simulink model "mvdc_KF_PointMassSep"  (R2018b)
settings: configuration reference "Active" (kept outside this file)
undefined symbols (not defined in the file): P_VDC_enableCovPropagation, P_VDC_ManualInitializationStartPose, P_VDC_ManualInitializationStateEstimation, P_VDC_measCov_GPS, P_VDC_measCov_velocity, P_VDC_measCov_VLOC, P_VDC_OutlierBounds, P_VDC_processCovVelocityFused, P_VDC_Var_ax_mps2, P_VDC_Var_ay_mps2, P_VDC_Var_yawRate_radps, P_VDC_YawAngleDepCovMode, res_dGPS_m, res_dPsi_radps, res_dVLOC_m, res_PsiGPS_rad, res_PsiVLOC_rad, res_sGPS_m, res_sVLOC_m, res_vx_mps, res_vy_mps, res_xGPS_m, res_xVLOC_m, res_yGPS_m, res_yVLOC_m, tS
libraries: rr_general x2
settings Model: DataDictionary=mvdc_KF.sldd  Creator=Madeline  LastModifiedBy=Kappertz

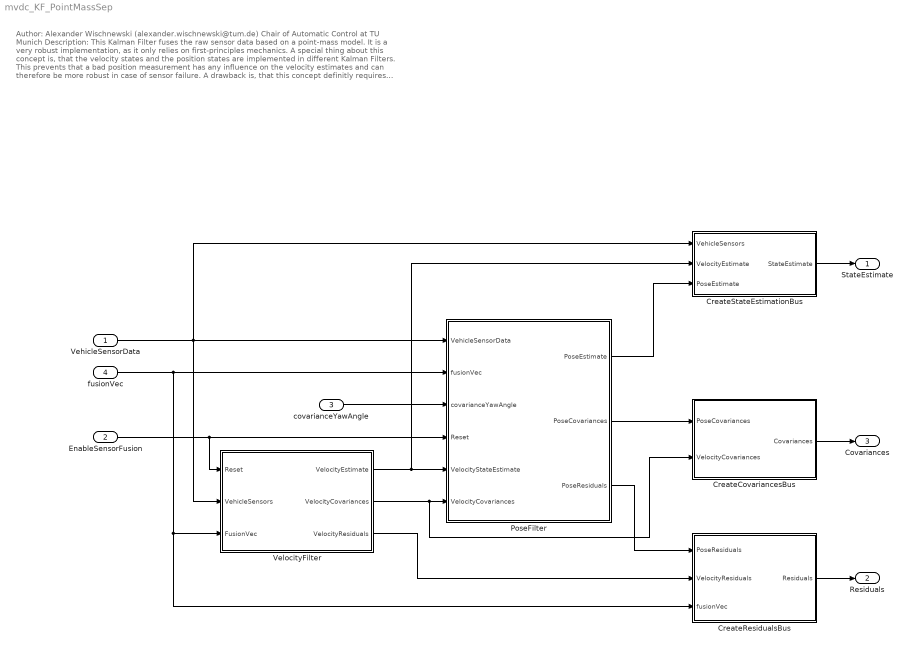
== system mvdc_KF_PointMassSep ==
  note: Author: Alexander Wischnewski (alexander.wischnewski@tum.de)
      | Chair of Automatic Control at TU Munich
      |
      | Description: This Kalman Filter fuses the raw sensor data based on a point-mass model. It is a very robust implementation, as it only relies on first-principles mechanics. A special thing about this concept is, that the velocity states and the position states are implemented in different Kalman Filters. This prevents that a bad position measurement has any influence on the velocity estimates and can therefore be more robust in case of sensor failure. A drawback is, that this concept definitly requires measurement of the vehicle-fixed velocities in lateral and longitudinal direction. Another drawback compared to a more complex vehicle model is, that it cannot filter the yaw rate as there are no derivative information about the yaw rate available. However, it is easy to tune and has comparable performance over the whole range of operating points.
      |
      | Inputs:
      | EnableSensorFusion Enable bit which activates the Kalman Filter
      | VehicleSensorData Raw sensor data
      | ActualPathOrientation Path orientation provided by the trajectory planner (used for weighting GPS and LIDAR via Covariance Matrix)
      | fusionVec Vector with bit-wise information about whether a sensor should be used for fusion or not
      |
      | Outputs:
      | StateEstimate Estimated state vector of the Kalman Filter
      | Residuals Pre-update measurement residuals of the Kalman Filter
      | Covariances Post-update Estimation Covariance Matrix of the Kalman Filter
  VehicleSensorData : Inport  OutDataTypeStr=Bus: VehicleSensorData
  EnableSensorFusion : Inport  Port=2  OutDataTypeStr=boolean
  covarianceYawAngle : Inport  Port=3
  fusionVec : Inport  Port=4  OutDataTypeStr=boolean  PortDimensions=9
  CreateCovariancesBus : Subsystem
  CreateResidualsBus : Subsystem
  CreateStateEstimationBus : Subsystem
  PoseFilter : Subsystem
  VelocityFilter : Subsystem
  "StateEstimate " : Outport  OutDataTypeStr=Bus: StateEstimation_state
  Residuals : Outport  Port=2  OutDataTypeStr=Bus: StateEstimation_residuals
  Covariances : Outport  Port=3  OutDataTypeStr=Bus: StateEstimation_covariances
  wires:
  CreateResidualsBus/1(Residuals) -> Residuals/1
  covarianceYawAngle/1 -> PoseFilter/3(covarianceYawAngle)
  EnableSensorFusion/1 -> VelocityFilter/1(Reset), PoseFilter/4(Reset)
  CreateCovariancesBus/1(Covariances) -> Covariances/1
  CreateStateEstimationBus/1(StateEstimate) -> "StateEstimate "/1
  VehicleSensorData/1 -> PoseFilter/1(VehicleSensorData), CreateStateEstimationBus/1(VehicleSensors), VelocityFilter/2(VehicleSensors)
  fusionVec/1 -> PoseFilter/2(fusionVec), VelocityFilter/3(FusionVec), CreateResidualsBus/3(fusionVec)
  VelocityFilter/1(VelocityEstimate) -> PoseFilter/5(VelocityStateEstimate), CreateStateEstimationBus/2(VelocityEstimate)
  VelocityFilter/2(VelocityCovariances) -> PoseFilter/6(VelocityCovariances), CreateCovariancesBus/2(VelocityCovariances)
  VelocityFilter/3(VelocityResiduals) -> CreateResidualsBus/2(VelocityResiduals)
  PoseFilter/1(PoseEstimate) -> CreateStateEstimationBus/3(PoseEstimate)
  PoseFilter/3(PoseResiduals) -> CreateResidualsBus/1(PoseResiduals)
  PoseFilter/2(PoseCovariances) -> CreateCovariancesBus/1(PoseCovariances)

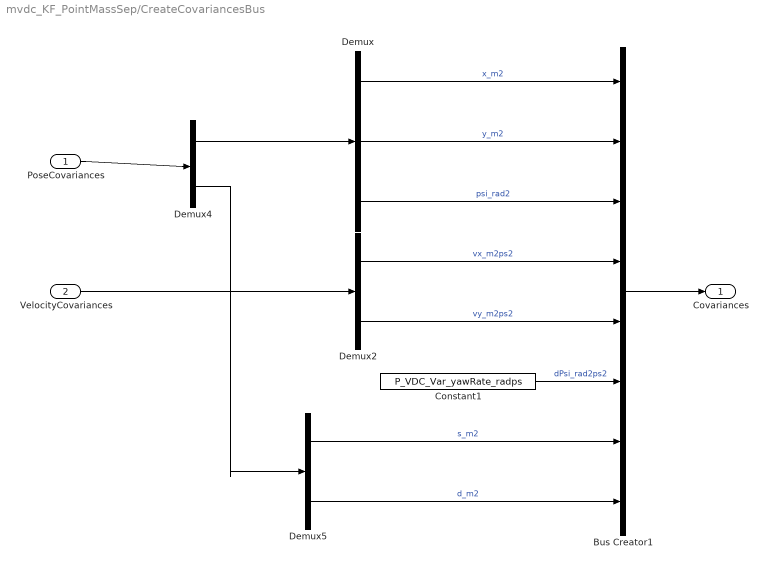
== system mvdc_KF_PointMassSep/CreateCovariancesBus ==
  PoseCovariances : Inport
  VelocityCovariances : Inport  Port=2
  Bus Creator1 : BusCreator  Inputs=8
  Constant1 : Constant  Value=P_VDC_Var_yawRate_radps
  Demux : Demux  Outputs=3
  Demux2 : Demux  Outputs=2
  Demux4 : Demux  Outputs=[3 2]
  Demux5 : Demux  Outputs=2
  Covariances : Outport
  wires:
  Bus Creator1/1 -> Covariances/1
  PoseCovariances/1 -> Demux4/1
  Demux/1 -> Bus Creator1/1  "x_m2"
  Demux/2 -> Bus Creator1/2  "y_m2"
  Demux/3 -> Bus Creator1/3  "psi_rad2"
  Demux2/1 -> Bus Creator1/4  "vx_m2ps2"
  Demux2/2 -> Bus Creator1/5  "vy_m2ps2"
  Constant1/1 -> Bus Creator1/6  "dPsi_rad2ps2"
  Demux5/1 -> Bus Creator1/7  "s_m2"
  Demux5/2 -> Bus Creator1/8  "d_m2"
  VelocityCovariances/1 -> Demux2/1
  Demux4/1 -> Demux/1
  Demux4/2 -> Demux5/1

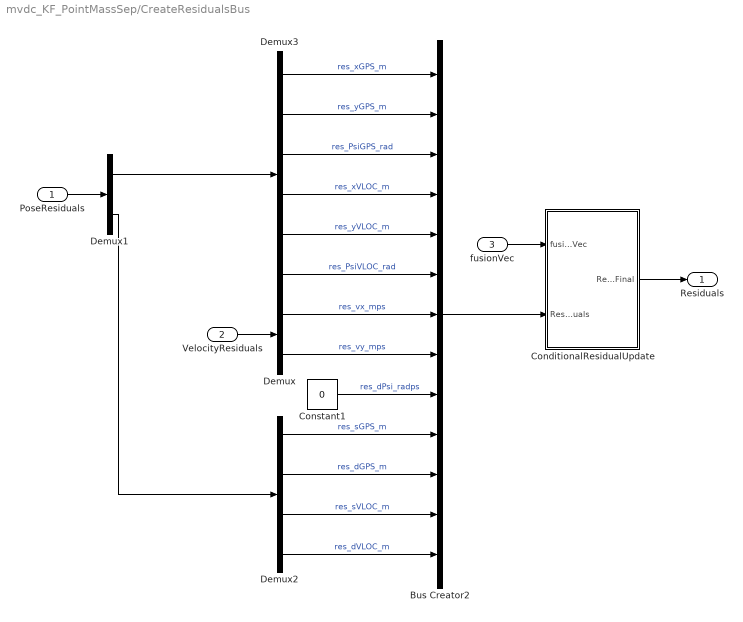
== system mvdc_KF_PointMassSep/CreateResidualsBus ==
  PoseResiduals : Inport
  VelocityResiduals : Inport  Port=2
  fusionVec : Inport  Port=3
  Bus Creator2 : BusCreator  Inputs=13
  ConditionalResidualUpdate : Subsystem
  Constant1 : Constant  Value=0
  Demux : Demux  Outputs=2
  Demux1 : Demux  Outputs=[6 4]
  Demux2 : Demux
  Demux3 : Demux  Outputs=6
  Residuals : Outport
  wires:
  Demux3/3 -> Bus Creator2/3  "res_PsiGPS_rad"
  Demux3/1 -> Bus Creator2/1  "res_xGPS_m"
  Demux3/2 -> Bus Creator2/2  "res_yGPS_m"
  Demux2/1 -> Bus Creator2/10  "res_sGPS_m"
  Demux2/2 -> Bus Creator2/11  "res_dGPS_m"
  Demux2/3 -> Bus Creator2/12  "res_sVLOC_m"
  Demux2/4 -> Bus Creator2/13  "res_dVLOC_m"
  fusionVec/1 -> ConditionalResidualUpdate/1(fusionVec)
  Bus Creator2/1 -> ConditionalResidualUpdate/2(Residuals)
  ConditionalResidualUpdate/1(ResidualsFinal) -> Residuals/1
  Demux3/4 -> Bus Creator2/4  "res_xVLOC_m"
  Demux3/5 -> Bus Creator2/5  "res_yVLOC_m"
  Demux3/6 -> Bus Creator2/6  "res_PsiVLOC_rad"
  Demux/1 -> Bus Creator2/7  "res_vx_mps"
  Demux/2 -> Bus Creator2/8  "res_vy_mps"
  Constant1/1 -> Bus Creator2/9  "res_dPsi_radps"
  VelocityResiduals/1 -> Demux/1
  PoseResiduals/1 -> Demux1/1
  Demux1/1 -> Demux3/1
  Demux1/2 -> Demux2/1

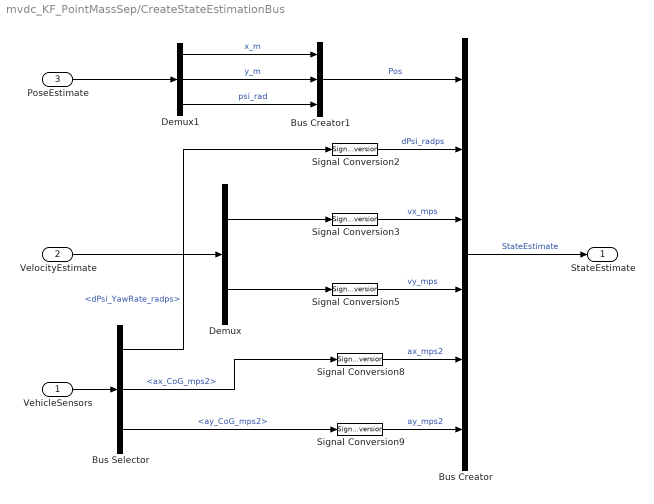
== system mvdc_KF_PointMassSep/CreateStateEstimationBus ==
  VehicleSensors : Inport
  VelocityEstimate : Inport  Port=2
  PoseEstimate : Inport  Port=3
  Bus Creator : BusCreator  Inputs=6
  Bus Creator1 : BusCreator  Inputs=3
  Bus Selector : BusSelector  OutputSignals=dPsi_YawRate_radps,ax_CoG_mps2,ay_CoG_mps2
  Demux : Demux  Outputs=2
  Demux1 : Demux  Outputs=3
  Signal Conversion{2..3,5,8..9} (5 alike) : SignalConversion  OverrideOpt=off
  StateEstimate : Outport
  wires:
  Bus Creator/1 -> StateEstimate/1  "StateEstimate"
  Signal Conversion3/1 -> Bus Creator/3  "vx_mps"
  Signal Conversion2/1 -> Bus Creator/2  "dPsi_radps"
  Signal Conversion5/1 -> Bus Creator/4  "vy_mps"
  Signal Conversion9/1 -> Bus Creator/6  "ay_mps2"
  Signal Conversion8/1 -> Bus Creator/5  "ax_mps2"
  VehicleSensors/1 -> Bus Selector/1
  Bus Selector/2 -> Signal Conversion8/1  "<ax_CoG_mps2>"
  Bus Selector/3 -> Signal Conversion9/1  "<ay_CoG_mps2>"
  Bus Selector/1 -> Signal Conversion2/1  "<dPsi_YawRate_radps>"
  VelocityEstimate/1 -> Demux/1
  Demux/1 -> Signal Conversion3/1
  Demux/2 -> Signal Conversion5/1
  PoseEstimate/1 -> Demux1/1
  Bus Creator1/1 -> Bus Creator/1  "Pos"
  Demux1/1 -> Bus Creator1/1  "x_m"
  Demux1/2 -> Bus Creator1/2  "y_m"
  Demux1/3 -> Bus Creator1/3  "psi_rad"

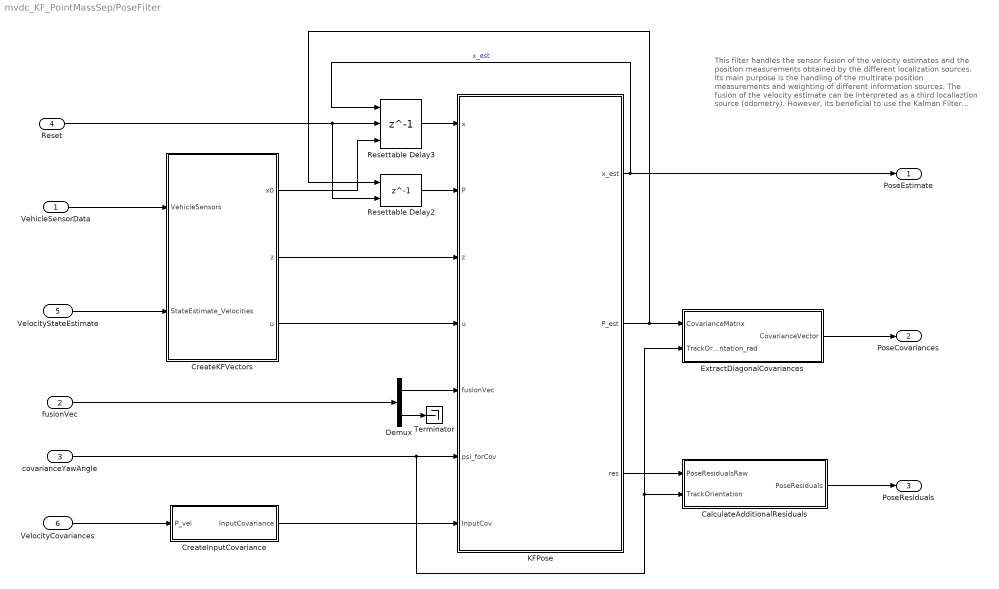
== system mvdc_KF_PointMassSep/PoseFilter ==
  note: This filter handles the sensor fusion
      | of the velocity estimates and the position measurements
      | obtained by the different localization sources. Its main purpose
      | is the handling of the multirate position measurements
      | and weighting of different information sources. The fusion
      | of the velocity estimate can be interpreted as a third localiaztion
      | source (odometry). However, its beneficial to use the Kalman Filter
      | framework here as the odometry drift is handled naturally therin.
  VehicleSensorData : Inport
  fusionVec : Inport  Port=2
  covarianceYawAngle : Inport  Port=3
  Reset : Inport  Port=4
  VelocityStateEstimate : Inport  Port=5
  VelocityCovariances : Inport  Port=6
  CalculateAdditionalResiduals : Subsystem
  CreateInputCovariance : Subsystem
  CreateKFVectors : Subsystem
  Demux : Demux  Outputs=[6 3]
  ExtractDiagonalCovariances : Subsystem
  KFPose : MATLAB Function  TreatAsAtomicUnit=on
  Resettable Delay2 : Delay  DelayLength=1  InitialCondition=eye(3)*0.1  ExternalReset=Rising
      settings: InputPortMap=u0,r5
  Resettable Delay3 : Delay  DelayLength=1  InitialConditionSource=Input port  ExternalReset=Rising
      settings: InputPortMap=u0,r5,p4
  Terminator : Terminator
  PoseEstimate : Outport
  PoseCovariances : Outport  Port=2
  PoseResiduals : Outport  Port=3
  wires:
  VelocityStateEstimate/1 -> CreateKFVectors/2(StateEstimate_Velocities)
  covarianceYawAngle/1 -> ExtractDiagonalCovariances/2(TrackOrientation_rad), CalculateAdditionalResiduals/2(TrackOrientation), KFPose/6(psi_forCov)
  Reset/1 -> Resettable Delay2/2, Resettable Delay3/2
  fusionVec/1 -> Demux/1
  VehicleSensorData/1 -> CreateKFVectors/1(VehicleSensors)
  VelocityCovariances/1 -> CreateInputCovariance/1(P_vel)
  KFPose/1(x_est) -> Resettable Delay3/1, PoseEstimate/1  "x_est"
  Resettable Delay3/1 -> KFPose/1(x)
  KFPose/2(P_est) -> ExtractDiagonalCovariances/1(CovarianceMatrix), Resettable Delay2/1
  Resettable Delay2/1 -> KFPose/2(P)
  Demux/1 -> KFPose/5(fusionVec)
  CreateKFVectors/1(x0) -> Resettable Delay3/3
  CreateInputCovariance/1(InputCovariance) -> KFPose/7(InputCov)
  Demux/2 -> Terminator/1
  CreateKFVectors/3(u) -> KFPose/4(u)
  CreateKFVectors/2(z) -> KFPose/3(z)
  CalculateAdditionalResiduals/1(PoseResiduals) -> PoseResiduals/1
  KFPose/3(res) -> CalculateAdditionalResiduals/1(PoseResidualsRaw)
  ExtractDiagonalCovariances/1(CovarianceVector) -> PoseCovariances/1

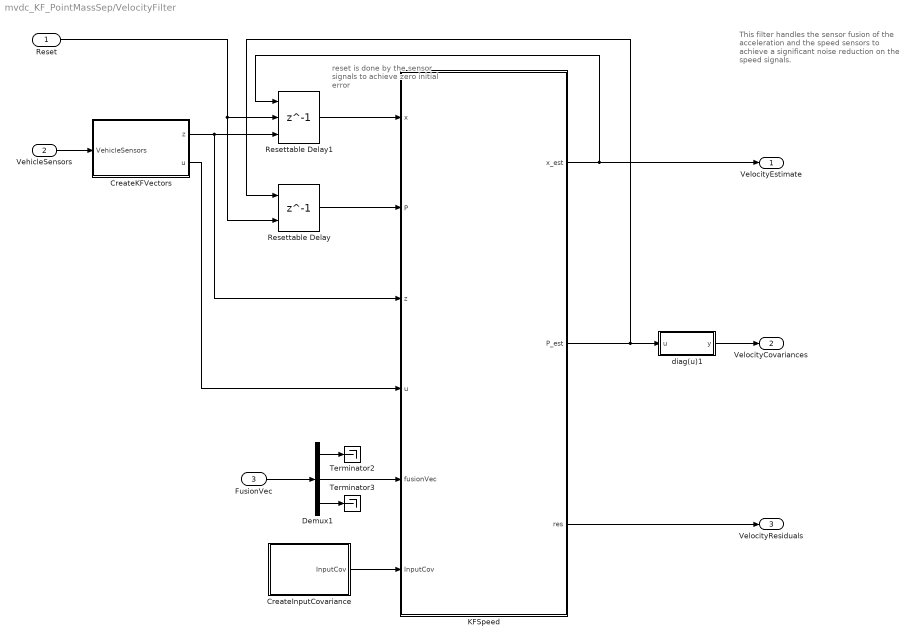
== system mvdc_KF_PointMassSep/VelocityFilter ==
  note: reset is done by
      | the sensor signals
      | to achieve zero
      | initial error
  note: This filter handles the sensor fusion
      | of the acceleration and the speed sensors
      | to achieve a significant noise reduction
      | on the speed signals.
  Reset : Inport
  VehicleSensors : Inport  Port=2
  FusionVec : Inport  Port=3
  CreateInputCovariance : Subsystem
  CreateKFVectors : Subsystem
  Demux1 : Demux  Outputs=[6 2 1]
  KFSpeed : MATLAB Function  TreatAsAtomicUnit=on
  Resettable Delay : Delay  DelayLength=1  DelayLengthUpperLimit=2  InitialCondition=eye(2)  ExternalReset=Rising
      settings: InputPortMap=u0,r5
  Resettable Delay1 : Delay  DelayLength=1  DelayLengthUpperLimit=2  InitialConditionSource=Input port  ExternalReset=Rising
      settings: InputPortMap=u0,r5,p4
  Terminator2 : Terminator
  Terminator3 : Terminator
  diag(u)1 : MATLAB Function  TreatAsAtomicUnit=on
  VelocityEstimate : Outport
  VelocityCovariances : Outport  Port=2
  VelocityResiduals : Outport  Port=3
  wires:
  Resettable Delay/1 -> KFSpeed/2(P)
  KFSpeed/1(x_est) -> Resettable Delay1/1, VelocityEstimate/1
  Resettable Delay1/1 -> KFSpeed/1(x)
  CreateKFVectors/1(z) -> Resettable Delay1/3, KFSpeed/3(z)
  KFSpeed/3(res) -> VelocityResiduals/1
  CreateKFVectors/2(u) -> KFSpeed/4(u)
  Demux1/2 -> KFSpeed/5(fusionVec)
  Demux1/3 -> Terminator3/1
  CreateInputCovariance/1(InputCov) -> KFSpeed/6(InputCov)
  Demux1/1 -> Terminator2/1
  FusionVec/1 -> Demux1/1
  Reset/1 -> Resettable Delay1/2, Resettable Delay/2
  VehicleSensors/1 -> CreateKFVectors/1(VehicleSensors)
  KFSpeed/2(P_est) -> diag(u)1/1(u), Resettable Delay/1
  diag(u)1/1(y) -> VelocityCovariances/1

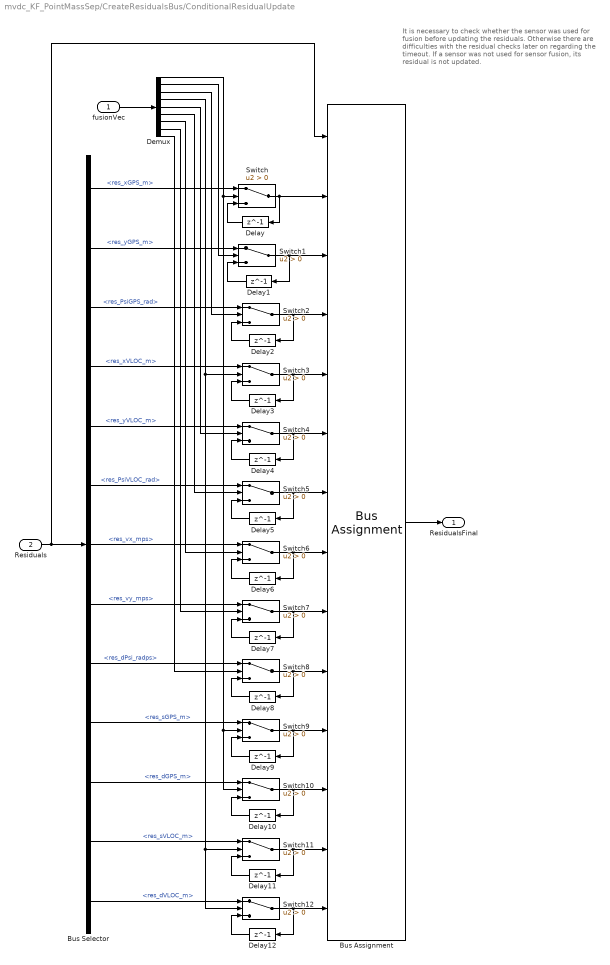
== system mvdc_KF_PointMassSep/CreateResidualsBus/ConditionalResidualUpdate ==
  note: It is necessary to check
      | whether the sensor was used for fusion
      | before updating the residuals. Otherwise
      | there are difficulties with the residual checks
      | later on regarding the timeout. If a sensor was
      | not used for sensor fusion, its residual is not updated.
  fusionVec : Inport
  Residuals : Inport  Port=2
  Bus Assignment : BusAssignment  AssignedSignals=res_xGPS_m,res_yGPS_m,res_PsiGPS_rad,res_xVLOC_m,res_yVLOC_m,res_PsiVLOC_rad,res_vx_mps,res_vy_mps,res_dPsi_radps,res_sGPS_m,res_dGPS_m,res_sVLOC_m,res_dVLOC_m
  Bus Selector : BusSelector  OutputSignals=res_xGPS_m,res_yGPS_m,res_PsiGPS_rad,res_xVLOC_m,res_yVLOC_m,res_PsiVLOC_rad,res_vx_mps,res_vy_mps,res_dPsi_radps,res_sGPS_m,res_dGPS_m,res_sVLOC_m,res_dVLOC_m
  Delay{,1..12} (13 alike) : Delay  DelayLength=1  InitialCondition=0
  Demux : Demux  Outputs=9
  Switch{,1..12} (13 alike) : Switch  Criteria=u2 > Threshold
  ResidualsFinal : Outport
  wires:
  Demux/5 -> Switch4/2
  Delay8/1 -> Switch8/3
  Switch8/1 -> Bus Assignment/10, Delay8/1
  Bus Selector/6 -> Switch5/1  "<res_PsiVLOC_rad>"
  Switch6/1 -> Bus Assignment/8, Delay6/1
  Delay6/1 -> Switch6/3
  Demux/7 -> Switch6/2
  Switch7/1 -> Bus Assignment/9, Delay7/1
  Delay7/1 -> Switch7/3
  Switch2/1 -> Bus Assignment/4, Delay2/1
  Switch4/1 -> Bus Assignment/6, Delay4/1
  Delay4/1 -> Switch4/3
  Delay/1 -> Switch/3
  Switch/1 -> Bus Assignment/2, Delay/1
  Bus Assignment/1 -> ResidualsFinal/1
  Demux/3 -> Switch2/2
  Residuals/1 -> Bus Assignment/1, Bus Selector/1
  Bus Selector/1 -> Switch/1  "<res_xGPS_m>"
  Demux/8 -> Switch7/2
  Demux/9 -> Switch8/2
  Delay5/1 -> Switch5/3
  Switch5/1 -> Bus Assignment/7, Delay5/1
  Demux/2 -> Switch1/2
  Demux/6 -> Switch5/2
  Demux/4 -> Switch12/2, Switch11/2, Switch3/2
  Bus Selector/8 -> Switch7/1  "<res_vy_mps>"
  Delay2/1 -> Switch2/3
  Bus Selector/7 -> Switch6/1  "<res_vx_mps>"
  Delay1/1 -> Switch1/3
  Bus Selector/2 -> Switch1/1  "<res_yGPS_m>"
  Switch1/1 -> Bus Assignment/3, Delay1/1
  fusionVec/1 -> Demux/1
  Delay3/1 -> Switch3/3
  Bus Selector/9 -> Switch8/1  "<res_dPsi_radps>"
  Switch12/1 -> Bus Assignment/14, Delay12/1
  Switch10/1 -> Bus Assignment/12, Delay10/1
  Switch11/1 -> Bus Assignment/13, Delay11/1
  Switch9/1 -> Bus Assignment/11, Delay9/1
  Bus Selector/10 -> Switch9/1  "<res_sGPS_m>"
  Delay9/1 -> Switch9/3
  Delay10/1 -> Switch10/3
  Delay11/1 -> Switch11/3
  Delay12/1 -> Switch12/3
  Bus Selector/13 -> Switch12/1  "<res_dVLOC_m>"
  Bus Selector/12 -> Switch11/1  "<res_sVLOC_m>"
  Bus Selector/11 -> Switch10/1  "<res_dGPS_m>"
  Demux/1 -> Switch/2, Switch10/2, Switch9/2
  Bus Selector/3 -> Switch2/1  "<res_PsiGPS_rad>"
  Bus Selector/4 -> Switch3/1  "<res_xVLOC_m>"
  Bus Selector/5 -> Switch4/1  "<res_yVLOC_m>"
  Switch3/1 -> Bus Assignment/5, Delay3/1

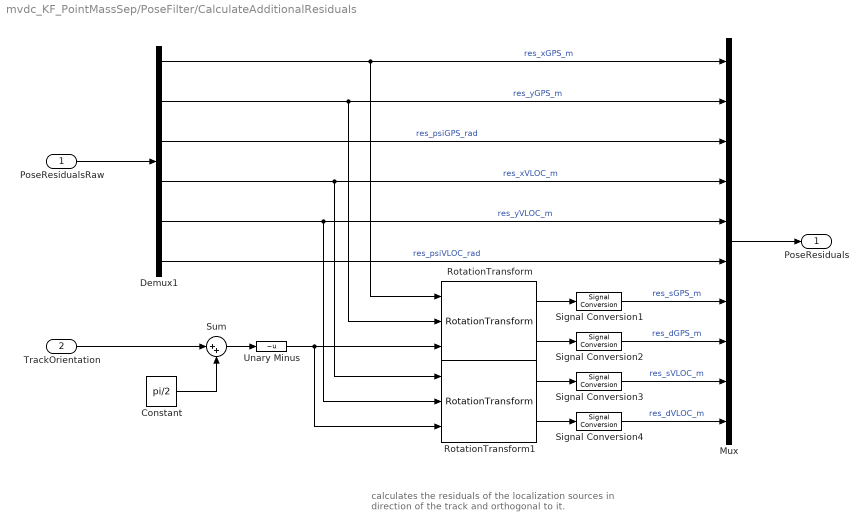
== system mvdc_KF_PointMassSep/PoseFilter/CalculateAdditionalResiduals ==
  note: calculates the residuals of the localization sources
      | in direction of the track and orthogonal to it.
  PoseResidualsRaw : Inport
  TrackOrientation : Inport  Port=2
  Constant : Constant  Value=pi/2
  Demux1 : Demux  Outputs=6
  Mux : Mux  Inputs=10
  RotationTransform : rr_general/RotationTransform  SystemSampleTime=-1
  RotationTransform1 : rr_general/RotationTransform  SystemSampleTime=-1
  Signal Conversion{1..4} (4 alike) : SignalConversion  OverrideOpt=off
  Sum : Sum  Inputs=|++
  Unary Minus : UnaryMinus
  PoseResiduals : Outport
  wires:
  Demux1/2 -> RotationTransform/2, Mux/2  "res_yGPS_m"
  RotationTransform/1 -> Signal Conversion1/1
  RotationTransform/2 -> Signal Conversion2/1
  RotationTransform1/2 -> Signal Conversion4/1
  RotationTransform1/1 -> Signal Conversion3/1
  Unary Minus/1 -> RotationTransform1/3, RotationTransform/3
  Constant/1 -> Sum/2
  Sum/1 -> Unary Minus/1
  Demux1/4 -> Mux/4, RotationTransform1/1  "res_xVLOC_m"
  Demux1/1 -> RotationTransform/1, Mux/1  "res_xGPS_m"
  Demux1/5 -> RotationTransform1/2, Mux/5  "res_yVLOC_m"
  Signal Conversion4/1 -> Mux/10  "res_dVLOC_m"
  Mux/1 -> PoseResiduals/1
  Signal Conversion3/1 -> Mux/9  "res_sVLOC_m"
  Signal Conversion2/1 -> Mux/8  "res_dGPS_m"
  Signal Conversion1/1 -> Mux/7  "res_sGPS_m"
  PoseResidualsRaw/1 -> Demux1/1
  TrackOrientation/1 -> Sum/1
  Demux1/3 -> Mux/3  "res_psiGPS_rad"
  Demux1/6 -> Mux/6  "res_psiVLOC_rad"

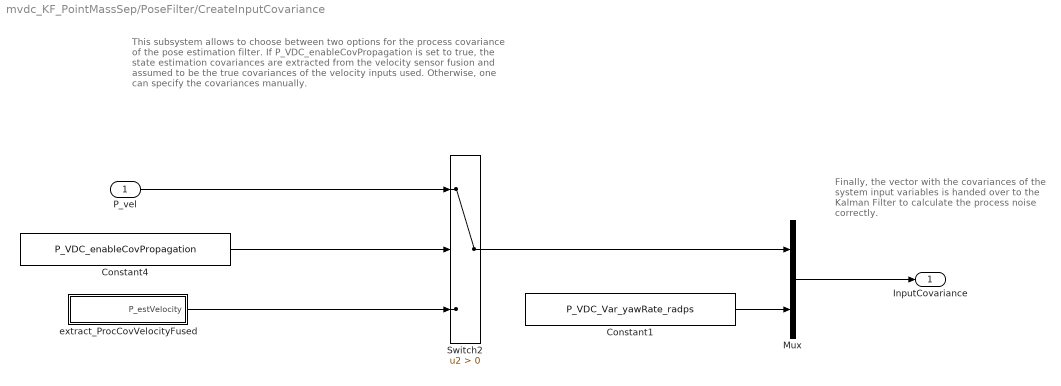
== system mvdc_KF_PointMassSep/PoseFilter/CreateInputCovariance ==
  note: Finally, the vector with the covariances
      | of the system input variables is handed over
      | to the Kalman Filter to calculate the
      | process noise correctly.
  note: This subsystem allows to choose between two options for the process
      | covariance of the pose estimation filter. If P_VDC_enableCovPropagation
      | is set to true, the state estimation covariances are extracted from the
      | velocity sensor fusion and assumed to be the true covariances of the
      | velocity inputs used. Otherwise, one can specify the covariances manually.
  P_vel : Inport
  Constant1 : Constant  Value=P_VDC_Var_yawRate_radps
  Constant4 : Constant  Value=P_VDC_enableCovPropagation
  Mux : Mux  Inputs=2
  Switch2 : Switch  Criteria=u2 > Threshold
  extract_ProcCovVelocityFused : Subsystem
  InputCovariance : Outport
  wires:
  extract_ProcCovVelocityFused/1(P_estVelocity) -> Switch2/3
  Constant4/1 -> Switch2/2
  Constant1/1 -> Mux/2
  Switch2/1 -> Mux/1
  Mux/1 -> InputCovariance/1
  P_vel/1 -> Switch2/1

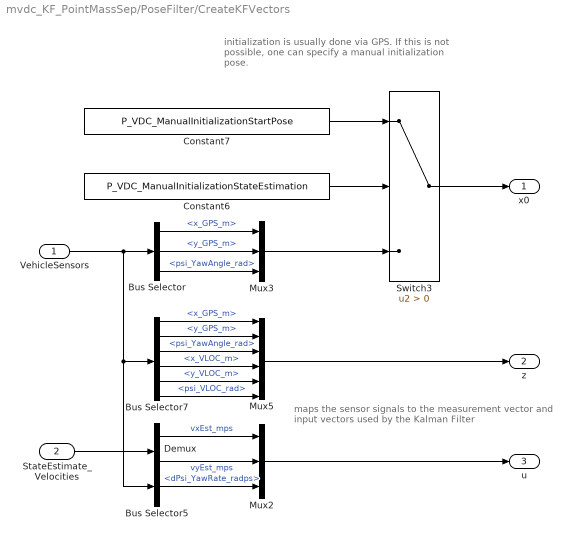
== system mvdc_KF_PointMassSep/PoseFilter/CreateKFVectors ==
  note: maps the sensor signals to the measurement vector
      | and input vectors used by the Kalman Filter
  note: initialization is usually done via GPS.
      | If this is not possible, one can specify a manual
      | initialization pose.
  VehicleSensors : Inport
  StateEstimate_Velocities : Inport  Port=2
  Bus Selector : BusSelector  OutputSignals=x_GPS_m,y_GPS_m,psi_YawAngle_rad
  Bus Selector5 : BusSelector  OutputSignals=dPsi_YawRate_radps
  Bus Selector7 : BusSelector  OutputSignals=x_GPS_m,y_GPS_m,psi_YawAngle_rad,x_VLOC_m,y_VLOC_m,psi_VLOC_rad
  Constant6 : Constant  Value=P_VDC_ManualInitializationStateEstimation
  Constant7 : Constant  Value=P_VDC_ManualInitializationStartPose
  Demux : Demux  Outputs=2
  Mux2 : Mux  Inputs=3
  Mux3 : Mux  Inputs=3
  Mux5 : Mux  Inputs=6
  Switch3 : Switch  Criteria=u2 > Threshold
  x0 : Outport
  z : Outport  Port=2
  u : Outport  Port=3
  wires:
  Mux2/1 -> u/1
  Bus Selector/1 -> Mux3/1  "<x_GPS_m>"
  Bus Selector/3 -> Mux3/3  "<psi_YawAngle_rad>"
  Bus Selector/2 -> Mux3/2  "<y_GPS_m>"
  Bus Selector7/1 -> Mux5/1  "<x_GPS_m>"
  Bus Selector7/2 -> Mux5/2  "<y_GPS_m>"
  Bus Selector7/3 -> Mux5/3  "<psi_YawAngle_rad>"
  Bus Selector7/4 -> Mux5/4  "<x_VLOC_m>"
  Bus Selector7/5 -> Mux5/5  "<y_VLOC_m>"
  Bus Selector7/6 -> Mux5/6  "<psi_VLOC_rad>"
  Mux5/1 -> z/1
  StateEstimate_Velocities/1 -> Demux/1
  Switch3/1 -> x0/1
  Mux3/1 -> Switch3/3
  Bus Selector5/1 -> Mux2/3  "<dPsi_YawRate_radps>"
  Constant6/1 -> Switch3/2
  Constant7/1 -> Switch3/1
  Demux/1 -> Mux2/1  "vxEst_mps"
  Demux/2 -> Mux2/2  "vyEst_mps"
  VehicleSensors/1 -> Bus Selector5/1, Bus Selector7/1, Bus Selector/1

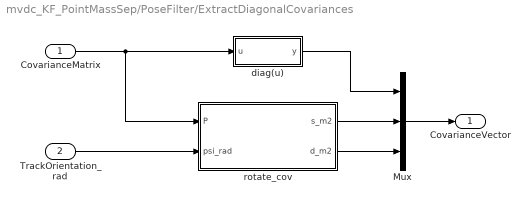
== system mvdc_KF_PointMassSep/PoseFilter/ExtractDiagonalCovariances ==
  CovarianceMatrix : Inport
  TrackOrientation_rad : Inport  Port=2
  Mux : Mux  Inputs=3
  diag(u) : MATLAB Function  TreatAsAtomicUnit=on
  rotate_cov : MATLAB Function  TreatAsAtomicUnit=on
  CovarianceVector : Outport
  wires:
  rotate_cov/2(d_m2) -> Mux/3
  diag(u)/1(y) -> Mux/1
  CovarianceMatrix/1 -> rotate_cov/1(P), diag(u)/1(u)
  TrackOrientation_rad/1 -> rotate_cov/2(psi_rad)
  Mux/1 -> CovarianceVector/1
  rotate_cov/1(s_m2) -> Mux/2

== system mvdc_KF_PointMassSep/VelocityFilter/CreateInputCovariance ==
  Constant : Constant  Value=P_VDC_Var_ax_mps2
  Constant1 : Constant  Value=P_VDC_Var_ay_mps2
  Constant2 : Constant  Value=P_VDC_Var_yawRate_radps
  Mux : Mux  Inputs=3
  InputCov : Outport
  wires:
  Constant/1 -> Mux/1
  Constant1/1 -> Mux/2
  Constant2/1 -> Mux/3
  Mux/1 -> InputCov/1

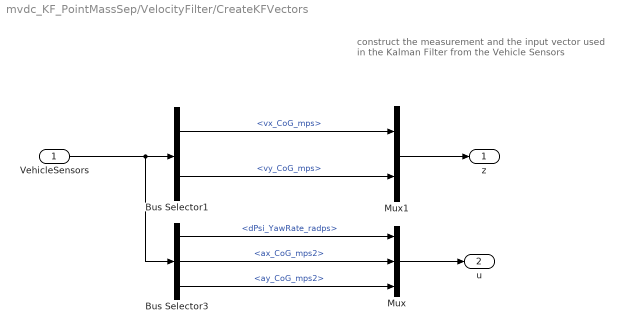
== system mvdc_KF_PointMassSep/VelocityFilter/CreateKFVectors ==
  note: construct the measurement and the input vector
      | used in the Kalman Filter from the Vehicle Sensors
  VehicleSensors : Inport
  Bus Selector1 : BusSelector  OutputSignals=vx_CoG_mps,vy_CoG_mps
  Bus Selector3 : BusSelector  OutputSignals=dPsi_YawRate_radps,ax_CoG_mps2,ay_CoG_mps2
  Mux : Mux  Inputs=3
  Mux1 : Mux  Inputs=2
  z : Outport
  u : Outport  Port=2
  wires:
  Mux1/1 -> z/1
  Mux/1 -> u/1
  Bus Selector3/3 -> Mux/3  "<ay_CoG_mps2>"
  Bus Selector1/2 -> Mux1/2  "<vy_CoG_mps>"
  Bus Selector1/1 -> Mux1/1  "<vx_CoG_mps>"
  Bus Selector3/1 -> Mux/1  "<dPsi_YawRate_radps>"
  VehicleSensors/1 -> Bus Selector3/1, Bus Selector1/1
  Bus Selector3/2 -> Mux/2  "<ax_CoG_mps2>"

== system mvdc_KF_PointMassSep/PoseFilter/CreateInputCovariance/extract_ProcCovVelocityFused ==
  Constant4 : Constant  Value=P_VDC_processCovVelocityFused
  P_estVelocity : Outport
  wires:
  Constant4/1 -> P_estVelocity/1

== matlab function mvdc_KF_PointMassSep/VelocityFilter/KFSpeed ==
  data: x input; P input; z input; u input; x_est output; P_est output; tS parameter; fusionVec input boolean size=2; InputCov input; res output; P_VDC_measCov_velocity parameter; P_VDC_OutlierBounds parameter
function [x_est, P_est, res] = KFSpeed(x, P, z, u, tS, fusionVec, InputCov,P_VDC_measCov_velocity, P_VDC_OutlierBounds)

[x_est, P_est, res]= kf_speed(x, z, u, tS, fusionVec, InputCov, P, P_VDC_measCov_velocity, P_VDC_OutlierBounds);

end

== matlab function mvdc_KF_PointMassSep/PoseFilter/KFPose ==
  data: x input; P input; z input; u input; fusionVec input boolean size=6; psi_forCov input; InputCov input; P_VDC_YawAngleDepCovMode parameter; x_est output; P_est output; P_VDC_measCov_GPS parameter; P_VDC_measCov_VLOC parameter; tS parameter; res output size=6; P_VDC_OutlierBounds parameter
 function [x_est, P_est, res] = KFPose(x, P, z, u, fusionVec, psi_forCov, InputCov, P_VDC_YawAngleDepCovMode, P_VDC_measCov_GPS, P_VDC_measCov_VLOC, tS, P_VDC_OutlierBounds)

[x_est, P_est, res] = kf_pose(x, z, u, fusionVec, psi_forCov, InputCov, P, P_VDC_YawAngleDepCovMode, P_VDC_measCov_GPS, P_VDC_measCov_VLOC, tS, P_VDC_OutlierBounds);


end

== matlab function mvdc_KF_PointMassSep/PoseFilter/ExtractDiagonalCovariances/diag(u) ==
  data: u input; y output
function y = diag(u)

y=diag(u);

% end

== matlab function mvdc_KF_PointMassSep/PoseFilter/ExtractDiagonalCovariances/rotate_cov ==
  data: P input; s_m2 output; psi_rad input; d_m2 output
function [s_m2, d_m2] = rotateCov(P, psi_rad)

% construct rotation matrix
R = [cos(psi_rad), -sin(psi_rad);...
  sin(psi_rad), cos(psi_rad)];

Prot = R*P(1:2, 1:2)*R';
Prot_diag = diag(Prot); 

s_m2 = Prot_diag(1); 
d_m2 = Prot_diag(2); 

% end

== matlab function mvdc_KF_PointMassSep/VelocityFilter/diag(u)1 ==
  data: u input; y output
function y = diag(u)

y=diag(u(1:2, 1:2));

% end
